simulink model "tank"  (R2015b)
settings: Solver=FixedStepDiscrete  StartTime=0.0  StopTime=inf  FixedStep=1e-3  RelTol=1e-3
libraries: sh_lib x74, nesl_utility x46, fl_lib x40, dspnetwork x33
(part 3 of 3)

== system tank/Virtual Gas Pipeline /The Gas Pipeline/Station 5 inlet valve ==
  valve : Inport
  Ball Valve : sh_lib/Valves/Flow Control Valves/Ball Valve  d_ball=18 in  d_orif=16 in  x_0=0 m  C_d=0.65  Re_cr=10  A_leak=1e-12 m^2
  Simulink-PS Converter : nesl_utility/Simulink-PS Converter  PhysicalDomain=network_engine_domain  SubClassName=ps_input  LeftPortType=input  RightPortType=output  PseudoPeriodic=off  Frequencies=[]  NoiseDistribution=none  NoiseParameters=[]  Unit=1  AffineConversion=off  InputFiltering=off  SimscapeFilterOrder=1  InputFilterTimeConstant=0.001  UdotUserProvided=1
  Inlet : PMIOPort  Port=1  Side=Left
  outlet : PMIOPort  Port=2  Side=Right
  wires:
  valve/1 -> Simulink-PS Converter/1
  connections:
  Simulink-PS Converter/RConn1 -- Ball Valve/LConn1
  Inlet/RConn1 -- Ball Valve/LConn2
  outlet/RConn1 -- Ball Valve/RConn1

== system tank/Virtual Gas Pipeline /The Gas Pipeline/Station 2 (With 3km pipeline)/Flow Measurement (KL//Hr) ==
  Constant : Constant  Value=3600
  Hydraulic Flow Rate Sensor : fl_lib/Hydraulic/Hydraulic Sensors/Hydraulic Flow Rate Sensor
  PS-Simulink Converter3 : nesl_utility/PS-Simulink Converter  PhysicalDomain=network_engine_domain  SubClassName=ps_output  LeftPortType=input  RightPortType=output  PseudoPeriodic=off  Frequencies=[]  Unit=m^3/s  AffineConversion=off
  Product : Product
  Inlet reference : PMIOPort  Port=1  Side=Left
  " Outlet Reference" : PMIOPort  Port=2  Side=Left
  Display out : Outport
  wires:
  Product/1 -> Display out/1
  Constant/1 -> Product/2
  PS-Simulink Converter3/1 -> Product/1
  connections:
  PS-Simulink Converter3/LConn1 -- Hydraulic Flow Rate Sensor/RConn1
  Hydraulic Flow Rate Sensor/RConn2 -- " Outlet Reference"/RConn1
  Hydraulic Flow Rate Sensor/LConn1 -- Inlet reference/RConn1

== system tank/Virtual Gas Pipeline /The Gas Pipeline/Station 2 (With 3km pipeline)/Measurement3 ==
  Hydraulic Reference3 : fl_lib/Hydraulic/Hydraulic Elements/Hydraulic Reference
  Ideal Hydraulic Pressure Sensor3 : fl_lib/Hydraulic/Hydraulic Sensors/Hydraulic Pressure Sensor
  PS-Simulink Converter3 : nesl_utility/PS-Simulink Converter  PhysicalDomain=network_engine_domain  SubClassName=ps_output  LeftPortType=input  RightPortType=output  PseudoPeriodic=off  Frequencies=[]  Unit=Pa  AffineConversion=off
  Port : PMIOPort  Port=1  Side=Left
  Display : Outport
  wires:
  PS-Simulink Converter3/1 -> Display/1
  connections:
  Ideal Hydraulic Pressure Sensor3/RConn1 -- Hydraulic Reference3/LConn1
  Ideal Hydraulic Pressure Sensor3/RConn2 -- PS-Simulink Converter3/LConn1
  Port/RConn1 -- Ideal Hydraulic Pressure Sensor3/LConn1

== system tank/Virtual Gas Pipeline /The Gas Pipeline/Station 3 (With 3km pipeline)/Flow Measurement (KL//Hr) ==
  Constant : Constant  Value=3600
  Hydraulic Flow Rate Sensor : fl_lib/Hydraulic/Hydraulic Sensors/Hydraulic Flow Rate Sensor
  PS-Simulink Converter3 : nesl_utility/PS-Simulink Converter  PhysicalDomain=network_engine_domain  SubClassName=ps_output  LeftPortType=input  RightPortType=output  PseudoPeriodic=off  Frequencies=[]  Unit=m^3/s  AffineConversion=off
  Product : Product
  Inlet reference : PMIOPort  Port=1  Side=Left
  " Outlet Reference" : PMIOPort  Port=2  Side=Left
  Display out : Outport
  wires:
  Product/1 -> Display out/1
  Constant/1 -> Product/2
  PS-Simulink Converter3/1 -> Product/1
  connections:
  PS-Simulink Converter3/LConn1 -- Hydraulic Flow Rate Sensor/RConn1
  Hydraulic Flow Rate Sensor/RConn2 -- " Outlet Reference"/RConn1
  Hydraulic Flow Rate Sensor/LConn1 -- Inlet reference/RConn1

== system tank/Virtual Gas Pipeline /The Gas Pipeline/Station 3 (With 3km pipeline)/Measurement2 ==
  Hydraulic Reference3 : fl_lib/Hydraulic/Hydraulic Elements/Hydraulic Reference
  Ideal Hydraulic Pressure Sensor3 : fl_lib/Hydraulic/Hydraulic Sensors/Hydraulic Pressure Sensor
  PS-Simulink Converter3 : nesl_utility/PS-Simulink Converter  PhysicalDomain=network_engine_domain  SubClassName=ps_output  LeftPortType=input  RightPortType=output  PseudoPeriodic=off  Frequencies=[]  Unit=Pa  AffineConversion=off
  Inlet : PMIOPort  Port=1  Side=Left
  Outlet : Outport
  wires:
  PS-Simulink Converter3/1 -> Outlet/1
  connections:
  Ideal Hydraulic Pressure Sensor3/RConn1 -- Hydraulic Reference3/LConn1
  Ideal Hydraulic Pressure Sensor3/RConn2 -- PS-Simulink Converter3/LConn1
  Inlet/RConn1 -- Ideal Hydraulic Pressure Sensor3/LConn1

== system tank/Virtual Gas Pipeline /The Gas Pipeline/Station 4 (With 3km pipeline)/Flow Measurement (KL//Hr) ==
  Constant : Constant  Value=3600
  Hydraulic Flow Rate Sensor : fl_lib/Hydraulic/Hydraulic Sensors/Hydraulic Flow Rate Sensor
  PS-Simulink Converter3 : nesl_utility/PS-Simulink Converter  PhysicalDomain=network_engine_domain  SubClassName=ps_output  LeftPortType=input  RightPortType=output  PseudoPeriodic=off  Frequencies=[]  Unit=m^3/s  AffineConversion=off
  Product : Product
  Inlet reference : PMIOPort  Port=1  Side=Left
  " Outlet Reference" : PMIOPort  Port=2  Side=Left
  Display out : Outport
  wires:
  Product/1 -> Display out/1
  Constant/1 -> Product/2
  PS-Simulink Converter3/1 -> Product/1
  connections:
  PS-Simulink Converter3/LConn1 -- Hydraulic Flow Rate Sensor/RConn1
  Hydraulic Flow Rate Sensor/RConn2 -- " Outlet Reference"/RConn1
  Hydraulic Flow Rate Sensor/LConn1 -- Inlet reference/RConn1

== system tank/Virtual Gas Pipeline /The Gas Pipeline/Station 4 (With 3km pipeline)/Measurement1 ==
  Hydraulic Reference3 : fl_lib/Hydraulic/Hydraulic Elements/Hydraulic Reference
  Ideal Hydraulic Pressure Sensor3 : fl_lib/Hydraulic/Hydraulic Sensors/Hydraulic Pressure Sensor
  PS-Simulink Converter3 : nesl_utility/PS-Simulink Converter  PhysicalDomain=network_engine_domain  SubClassName=ps_output  LeftPortType=input  RightPortType=output  PseudoPeriodic=off  Frequencies=[]  Unit=Pa  AffineConversion=off
  Port : PMIOPort  Port=1  Side=Left
  Display : Outport
  wires:
  PS-Simulink Converter3/1 -> Display/1
  connections:
  Ideal Hydraulic Pressure Sensor3/RConn1 -- Hydraulic Reference3/LConn1
  Ideal Hydraulic Pressure Sensor3/RConn2 -- PS-Simulink Converter3/LConn1
  Port/RConn1 -- Ideal Hydraulic Pressure Sensor3/LConn1

== system tank/Virtual Gas Pipeline /The Gas Pipeline/Station 5 (With 3km pipeline)/Flow Measurement (KL//Hr) ==
  Constant : Constant  Value=3600
  Hydraulic Flow Rate Sensor : fl_lib/Hydraulic/Hydraulic Sensors/Hydraulic Flow Rate Sensor
  PS-Simulink Converter3 : nesl_utility/PS-Simulink Converter  PhysicalDomain=network_engine_domain  SubClassName=ps_output  LeftPortType=input  RightPortType=output  PseudoPeriodic=off  Frequencies=[]  Unit=m^3/s  AffineConversion=off
  Product : Product
  Inlet reference : PMIOPort  Port=1  Side=Left
  " Outlet Reference" : PMIOPort  Port=2  Side=Left
  Display out : Outport
  wires:
  Product/1 -> Display out/1
  Constant/1 -> Product/2
  PS-Simulink Converter3/1 -> Product/1
  connections:
  PS-Simulink Converter3/LConn1 -- Hydraulic Flow Rate Sensor/RConn1
  Hydraulic Flow Rate Sensor/RConn2 -- " Outlet Reference"/RConn1
  Hydraulic Flow Rate Sensor/LConn1 -- Inlet reference/RConn1

== system tank/Virtual Gas Pipeline /The Gas Pipeline/Station 5 (With 3km pipeline)/Measurement6 ==
  Hydraulic Reference3 : fl_lib/Hydraulic/Hydraulic Elements/Hydraulic Reference
  Ideal Hydraulic Pressure Sensor3 : fl_lib/Hydraulic/Hydraulic Sensors/Hydraulic Pressure Sensor
  PS-Simulink Converter3 : nesl_utility/PS-Simulink Converter  PhysicalDomain=network_engine_domain  SubClassName=ps_output  LeftPortType=input  RightPortType=output  PseudoPeriodic=off  Frequencies=[]  Unit=Pa  AffineConversion=off
  Port : PMIOPort  Port=1  Side=Left
  Display : Outport
  wires:
  PS-Simulink Converter3/1 -> Display/1
  connections:
  Ideal Hydraulic Pressure Sensor3/RConn1 -- Hydraulic Reference3/LConn1
  Ideal Hydraulic Pressure Sensor3/RConn2 -- PS-Simulink Converter3/LConn1
  Port/RConn1 -- Ideal Hydraulic Pressure Sensor3/LConn1
